simulink model "Stimulation_Cerebrale"  (R2020b)
settings: Solver=VariableStepAuto  StartTime=0.0  StopTime=10.0  RelTol=1e-3
values from neighbouring files (symbols this model uses):
  Atilde = [(-1+mu1*z1*(1-z1/m1)*c11), -mu1*z1*(1-z1/m1)*c12 ... (first row only)    [Analyse_Stimulation_Cerebrale_Corrige.m]
  Btilde = [a*mu1*z1*(1-z1/m1); 0]    [Analyse_Stimulation_Cerebrale_Corrige.m]
  K = K_LQI(1:2)    [Analyse_Robustesse_LQI_Corrige.m]    (also in Analyse_Stimulation_Cerebrale_Corrige.m = [0.28, -0.54])
  M = 0.11    [Analyse_Stimulation_Cerebrale_Corrige.m]
  tau1 = 0.015    [Analyse_Stimulation_Cerebrale_Corrige.m]
  tau2 = 0.03    [Analyse_Stimulation_Cerebrale_Corrige.m]
settings Model: Creator=Sandou  LastModifiedBy=Sandou

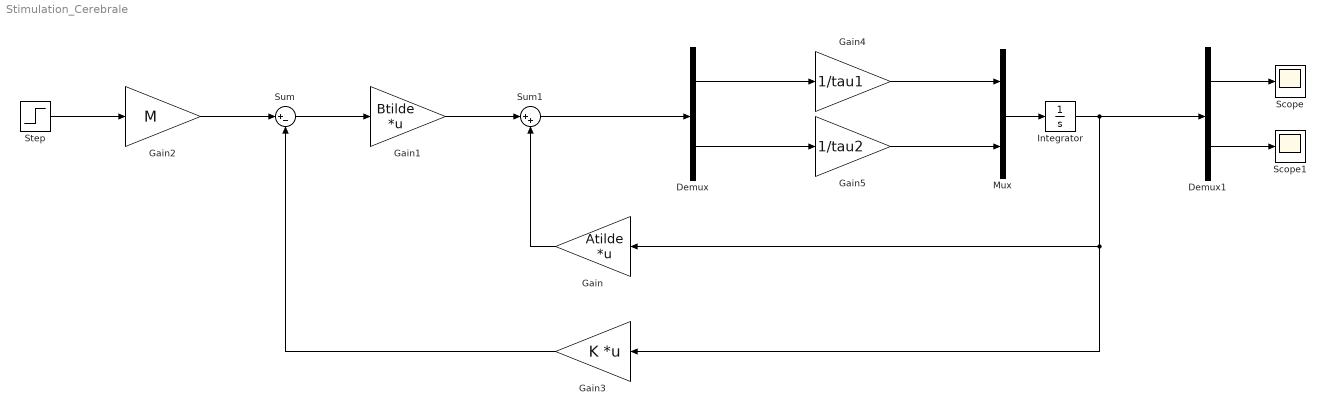
== system Stimulation_Cerebrale ==
  Demux : Demux  Outputs=2
  Demux1 : Demux  Outputs=2
  Gain : Gain  Gain=Atilde  Multiplication=Matrix(K*u)
  Gain1 : Gain  Gain=Btilde  Multiplication=Matrix(K*u)
  Gain2 : Gain  Gain=M
  Gain3 : Gain  Gain=K  Multiplication=Matrix(K*u)
  Gain4 : Gain  Gain=1/tau1
  Gain5 : Gain  Gain=1/tau2
  Integrator : Integrator
  Mux : Mux  Inputs=2
  Scope : Scope
  Scope1 : Scope
  Step : Step  SampleTime=0
  Sum : Sum  Inputs=|+-
  Sum1 : Sum  Inputs=|++
  wires:
  Gain2/1 -> Sum/1
  Gain3/1 -> Sum/2
  Sum/1 -> Gain1/1
  Integrator/1 -> Demux1/1, Gain/1, Gain3/1
  Demux/2 -> Gain5/1
  Demux/1 -> Gain4/1
  Mux/1 -> Integrator/1
  Gain4/1 -> Mux/1
  Gain5/1 -> Mux/2
  Step/1 -> Gain2/1
  Demux1/1 -> Scope/1
  Demux1/2 -> Scope1/1
  Gain/1 -> Sum1/2
  Gain1/1 -> Sum1/1
  Sum1/1 -> Demux/1
